simulink model "Old Segmentation"  (R2021a)
settings: Solver=VariableStepAuto  StartTime=0.0  StopTime=10.0  RelTol=1e-3
undefined symbols (not defined in the file): Sim3dSensor
libraries: visionsinks x3, simulink x2, sim3dcameralib x1, sim3dlib x1, uavsim3dlib x1
settings DebuggingCC: UnconnectedInputMsg=none  UnconnectedOutputMsg=none  UnconnectedLineMsg=none
settings ModelReferenceCC: EnableRefExpFcnMdlSchedulingChecks=off
settings RTWCC: Description=Generic Real-Time Target  GPUComputeCapability=5.0  DLArmComputeVersion=20.02.1

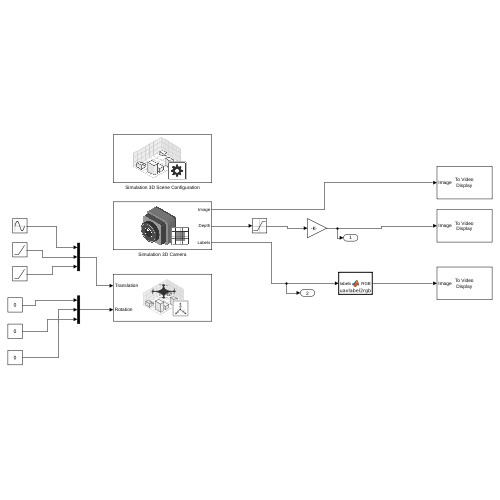
[thumbnail: Simulink's stored preview of the top-level diagram]
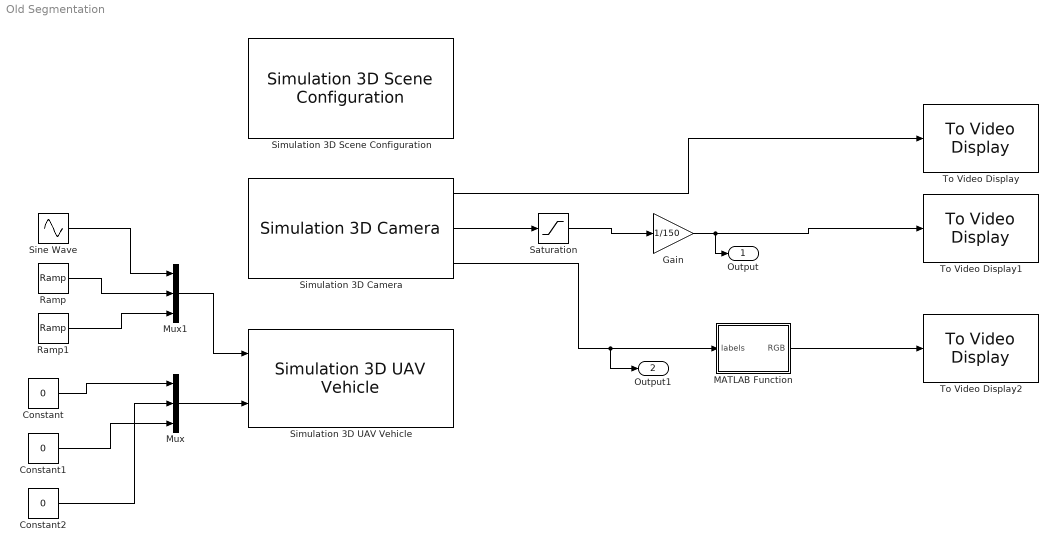
== system Old Segmentation ==
  Constant : Constant  Value=0
  Constant1 : Constant  Value=0
  Constant2 : Constant  Value=0
  Gain : Gain  Gain=1/150
  MATLAB Function : MATLAB Function  TreatAsAtomicUnit=on
  Mux : Mux  Inputs=3
  Mux1 : Mux  Inputs=3
  Ramp : simulink/Sources/Ramp  slope=1  start=0  InitialOutput=0
  Ramp1 : simulink/Sources/Ramp  slope=1  start=0  InitialOutput=0
  Saturation : Saturate
  Simulation 3D Camera : sim3dcameralib/Simulation 3D Camera  Priority=1  sensorTag=Sim3dSensor�  sensorId=1  sensorName=Sim3dSensor�  vehTagList={'Scene Origin';'SimulinkVehicle1'}  vehTag=Scene Origin  mountLoc=Origin  offsetFlag=on  tmountOffset=[0, 0, 0]  rmountOffset=[0, 0, 0]  FocalLength=[1109, 1109]  OpticalCenter=[640, 360]  ImageSize=[720, 1280]  RadialDistortion=[0, 0]  TangentialDistortion=[0, 0]  SensorSkew=0  DepthOutportEnabled=on  SemanticOutportEnabled=on  TransformOutportEnabled=off  SampleTime=-1  mountPoint=[0 0 0]  mountOrientation=[0 0 0]  aMode=4  ID=1
  Simulation 3D Scene Configuration : sim3dlib/Simulation 3D Scene Configuration  Priority=0  ProjectFormat=Default Scenes  SceneDesc=US city block  ProjectName=/MATLAB/toolbox/shared/sim3d_projects/automotive_project_linux/UE/LinuxNoEditor/VehicleSimulation.sh  ScenePath=/Game/Maps/USCityBlock  EnableOpenDRIVE=off  vehTagList={'Scene Origin'}  vehTag=Scene Origin  FreeCameraInitialTranslation=[0, 0, 0]  FreeCameraDefaultInitialTranslation=[-6, 0, 2]  FreeCameraInitialRotation=[0, 0, 0]  FreeCameraDefaultInitialRotation=[0, -15, 0]  OpVisEn=off  Ts=1/60  EnableWindow=on  EnableRemoteAccess=off  EnableWeather=off  SunAzimuth=90  SunAltitude=40.0  wind=1  clouds=10  fog=0  rain=0  UseTrueOrigin=off  sensorTag=MainCamera1  sensorId=1  sensorName=MainCamera1  mountLoc=Origin  offsetFlag=off  tmountOffset=[0, 0, 0]  rmountOffset=[0, 0, 0]  HorizontalResolution=1280  VerticalResolution=720  HorizontalFOV=60  mountPoint=[0 0 0]  mountOrientation=[0 0 0]  aMode=4  ID=1  GeoTrigger=Inactive
  Simulation 3D UAV Vehicle : uavsim3dlib/Simulation 3D UAV Vehicle  Priority=-1  Mesh=Quadrotor  MeshPath=/MathWorksUAVContent/UAVs/HexaRotorUAV/HexaRotor.HexaRotor  Color=Black  ActorName=SimulinkVehicle1  UseGlobalFrame=off  InitialTranslation=[0 0 0]  InitialRotation=[0 0 0]  InitialTranslationGlobal=[0 0 0]  InitialGeoOrigin=[0 0 0]  InitialRotationGlobal=[0 0 0]  SampleTime=-1  ActorType=SimulinkVehicle  ID=1  aMode=4  ActorTag=SimulinkVehicle1
  Sine Wave : Sin  SampleTime=0
  To Video Display : visionsinks/To Video Display  windowSizeMode=Normal  openAtMdlStart=on  fullScreen=off  videoWindowX=536805376  videoWindowY=536805376  saveWindowSize=off  videoWindowWidth=2147483647  videoWindowHeight=2147483647  inputColorFormat=RGB  inputType=Obsolete  imagePorts=One multidimensional signal  OutputDevice=On-screen video monitor  dataOrg=Column-major  isWindowOpen=off
  To Video Display1 : visionsinks/To Video Display  windowSizeMode=Normal  openAtMdlStart=on  fullScreen=off  videoWindowX=536805376  videoWindowY=536805376  saveWindowSize=off  videoWindowWidth=2147483647  videoWindowHeight=2147483647  inputColorFormat=RGB  inputType=Obsolete  imagePorts=One multidimensional signal  OutputDevice=On-screen video monitor  dataOrg=Column-major  isWindowOpen=off
  To Video Display2 : visionsinks/To Video Display  windowSizeMode=Normal  openAtMdlStart=on  fullScreen=off  videoWindowX=536805376  videoWindowY=536805376  saveWindowSize=off  videoWindowWidth=2147483647  videoWindowHeight=2147483647  inputColorFormat=RGB  inputType=Obsolete  imagePorts=One multidimensional signal  OutputDevice=On-screen video monitor  dataOrg=Column-major  isWindowOpen=off
  Output : Outport
  Output1 : Outport  Port=2
  wires:
  Mux/1 -> Simulation 3D UAV Vehicle/2
  Constant/1 -> Mux/1
  Constant1/1 -> Mux/3
  Constant2/1 -> Mux/2
  Sine Wave/1 -> Mux1/1
  Ramp/1 -> Mux1/2
  Ramp1/1 -> Mux1/3
  Mux1/1 -> Simulation 3D UAV Vehicle/1
  Simulation 3D Camera/1 -> To Video Display/1
  Simulation 3D Camera/2 -> Saturation/1
  MATLAB Function/1(RGB) -> To Video Display2/1
  Simulation 3D Camera/3 -> Output1/1, MATLAB Function/1(labels)
  Saturation/1 -> Gain/1
  Gain/1 -> Output/1, To Video Display1/1

== matlab function Old Segmentation/MATLAB Function ==
  data: labels input; RGB output


function RGB = uavlabel2rgb(labels)
coder.extrinsic('label2rgb');
RGB = coder.nullcopy(zeros(size(labels,1),size(labels,2),3,class(labels)));
cmap = sim3dColormap;
RGB = label2rgb(labels, cmap);
end

function cmap = sim3dColormap
cmap = [
128 0 0
0 0 0 
72 0 90
0 0 0
192 192 192
128 0 128
128 64 128
60 40 222
128 128 0
64 0 128
0 0 0
192 128 128
192 128 128
192 128 128
192 128 128
192 128 128
0 0 0
0 0 0
192 128 128
192 128 128
192 128 128
0 0 0
192 128 128
0 0 0
192 128 128
0 0 0 
0 0 0
0 0 0
0 0 0
0 0 0
0 0 0
0 0 0
0 0 0
0 0 0 
0 0 0 
0 0 0
0 0 0
0 0 0
192 128 128
0 0 0
192 128 128
129 129 128
192 128 128
192 128 128
0 0 0
0 0 0
0 0 0
192 128 128
192 128 128
192 128 128 
192 128 128
192 128 128
192 128 128
0 0 0
0 0 0
0 0 0
128 128 128
60 40 128
60 40 128
60 40 128
0 0 0
0 0 0 
0 0 0
0 0 0
0 0 0
0 0 0
240 150 25
0 0 0
0 0 0
0 0 0
150 50 15
0 128 192
];

cmap = cmap ./ 255;
end
